simulink model "project 3 - RLS"  (R2018b)
settings: Solver=VariableStepAuto  StartTime=0.0  StopTime=1000  RelTol=1e-3
undefined symbols (not defined in the file): d, m, tmp
libraries: commchan3 x1
settings Model: Creator=DearUser  LastModifiedBy=DearUser

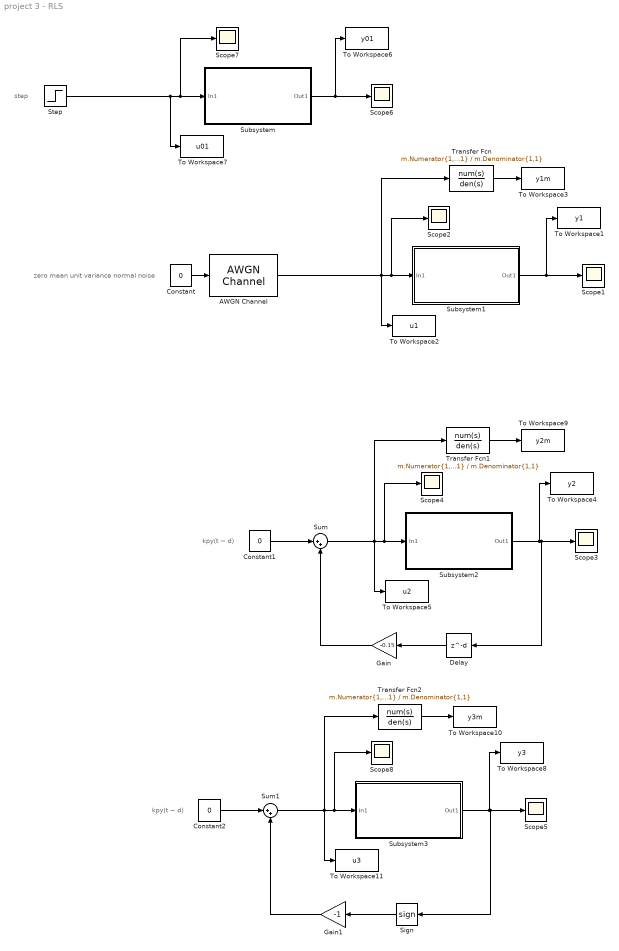
== system project 3 - RLS ==
  note: step
  note: zero mean unit variance normal noise
  note: kpy(t − d)
  note: kpy(t − d)
  AWGN Channel : commchan3/AWGN Channel  InputProcessing=Columns as channels (frame based)  seed=67  noiseMode=Variance from mask  EbNodB=10  EsNodB=10  SNRdB=10  bitsPerSym=1  Ps=1  Tsym=1  variance=1
      settings: SourceProductName=Communications Toolbox
  Constant : Constant  Value=0
  Constant1 : Constant  Value=0
  Constant2 : Constant  Value=0
  Delay : Delay  DelayLength=d
  Gain : Gain  Gain=-0.15
  Gain1 : Gain  Gain=-1
  Scope{1..8} (8 alike) : Scope
  Sign : Signum
  Step : Step  Time=100  SampleTime=0
  Subsystem : Subsystem  mask{sfcnParam1=tmp}
      mask prompts: sfcnParam1 "tmp:"
      mask help: Simulink:masks:GenSFuncDesc_MD
      mask Help: eval('feval(''rtwprivate'',''rtwhelpview'',''rtw_sfcn_block'')');
  Subsystem1 : Subsystem  mask{sfcnParam1=tmp}
      mask prompts: sfcnParam1 "tmp:"
      mask help: Simulink:masks:GenSFuncDesc_MD
      mask Help: eval('feval(''rtwprivate'',''rtwhelpview'',''rtw_sfcn_block'')');
  Subsystem2 : Subsystem  mask{sfcnParam1=tmp}
      mask prompts: sfcnParam1 "tmp:"
      mask help: Simulink:masks:GenSFuncDesc_MD
      mask Help: eval('feval(''rtwprivate'',''rtwhelpview'',''rtw_sfcn_block'')');
  Subsystem3 : Subsystem  mask{sfcnParam1=tmp}
      mask prompts: sfcnParam1 "tmp:"
      mask help: Simulink:masks:GenSFuncDesc_MD
      mask Help: eval('feval(''rtwprivate'',''rtwhelpview'',''rtw_sfcn_block'')');
  Sum : Sum  Inputs=|++
  Sum1 : Sum  Inputs=|++
  To Workspace1 : ToWorkspace  VariableName=y1  SaveFormat=Timeseries  SampleTime=-1
  To Workspace10 : ToWorkspace  VariableName=y3m  SaveFormat=Timeseries  SampleTime=-1
  To Workspace11 : ToWorkspace  VariableName=u3  SaveFormat=Timeseries  SampleTime=-1
  To Workspace2 : ToWorkspace  VariableName=u1  SaveFormat=Timeseries  SampleTime=-1
  To Workspace3 : ToWorkspace  VariableName=y1m  SaveFormat=Timeseries  SampleTime=-1
  To Workspace4 : ToWorkspace  VariableName=y2  SaveFormat=Timeseries  SampleTime=-1
  To Workspace5 : ToWorkspace  VariableName=u2  SaveFormat=Timeseries  SampleTime=-1
  To Workspace6 : ToWorkspace  VariableName=y01  SaveFormat=Timeseries  SampleTime=-1
  To Workspace7 : ToWorkspace  VariableName=u01  SaveFormat=Timeseries  SampleTime=-1
  To Workspace8 : ToWorkspace  VariableName=y3  SaveFormat=Timeseries  SampleTime=-1
  To Workspace9 : ToWorkspace  VariableName=y2m  SaveFormat=Timeseries  SampleTime=-1
  Transfer Fcn : TransferFcn  Numerator=m.Numerator{1,1}  Denominator=m.Denominator{1,1}
  Transfer Fcn1 : TransferFcn  Numerator=m.Numerator{1,1}  Denominator=m.Denominator{1,1}
  Transfer Fcn2 : TransferFcn  Numerator=m.Numerator{1,1}  Denominator=m.Denominator{1,1}
  wires:
  Subsystem/1(Out1) -> To Workspace6/1, Scope6/1
  Step/1 -> To Workspace7/1, Subsystem/1(In1), Scope7/1
  Constant/1 -> AWGN Channel/1
  AWGN Channel/1 -> To Workspace2/1, Subsystem1/1(In1), Scope2/1, Transfer Fcn/1
  Subsystem1/1(Out1) -> To Workspace1/1, Scope1/1
  Transfer Fcn/1 -> To Workspace3/1
  Constant1/1 -> Sum/1
  Delay/1 -> Gain/1
  Subsystem2/1(Out1) -> To Workspace4/1, Delay/1, Scope3/1
  Gain/1 -> Sum/2
  Transfer Fcn1/1 -> To Workspace9/1
  Sum/1 -> Transfer Fcn1/1, Subsystem2/1(In1), Scope4/1, To Workspace5/1
  Transfer Fcn2/1 -> To Workspace10/1
  Sign/1 -> Gain1/1
  Gain1/1 -> Sum1/2
  Subsystem3/1(Out1) -> To Workspace8/1, Sign/1, Scope5/1
  Constant2/1 -> Sum1/1
  Sum1/1 -> To Workspace11/1, Subsystem3/1(In1), Scope8/1, Transfer Fcn2/1

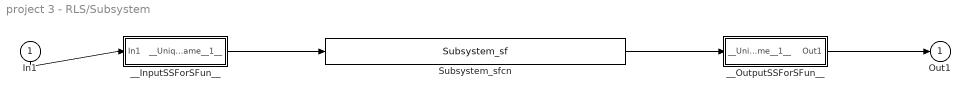
== system project 3 - RLS/Subsystem ==
  In1 : Inport
  Subsystem_sfcn : S-Function  FunctionName=Subsystem_sf  Parameters=sfcnParam1  SFunctionModules=""  SFunctionDeploymentMode=off  EnableBusSupport=off  mask{rtw_sf_name=Subsystem_sf, showVar=off, sfcnParam1=sfcnParam1}
      mask prompts: rtw_sf_name "Simulink:masks:GenSFuncName_MP"; showVar "Simulink:masks:GenSFuncShowModuleList_MP"; sfcnParam1 "tmp:"
      mask help: Simulink:masks:GenSFuncDesc_MD
      mask init:
      | displist = '';
      | if ~strcmp(get_param(gcb, 'FunctionName'), rtw_sf_name);
      |   set_param(gcb, 'FunctionName', rtw_sf_name);
      | end
      | % Check if we are generating code
      | rtw_mode = false;
      | if strcmpi(get_param(bdroot(gcb),'SimulationStatus'),'Initializing')
      | 	rtw_mode = strcmpi(get_param(bdroot(gcb),'BuildingRTWCode'),'on') && ...
      | 		~strcmpi(get_param(bdroot(gcb),'TargetStyle'),'SimulationTarget');
      | end
      | if showVar || rtw_mode
      | 	if exist('rtwsfunc') == 2 | exist('rtwsfunc') == 6
      | 		tmplist = rtwsfunc(rtw_sf_name,gcb);
      | 		tmplist = DAStudio.message('Simulink:masks:GenSFuncListOfModules_IC', tmplist);
      | 	elseif showVar
      | 		tmplist1 = DAStudio.message('Simulink:masks:GenSFuncListOfModules_IC', '');
      |         tmplist2 = DAStudio.message('Simulink:masks:GenSFuncNotLicensed_IC');
      |         tmplist = [tmplist1 tmplist2];
      |  	end
      | end
      | if showVar
      |   displist = tmplist;
      | end
      settings: CopyFcn=|
      | if ~strcmp(get_param(gcb,'Linkstatus'),'none') && ...
      | ~strcmp(get_param(gcb,'Linkstatus'),'implicit')
      |   set_param(gcb,'LinkStatus','none');
      | end
      mask Help: eval('feval(''rtwprivate'',''rtwhelpview'',''rtw_sfcn_block'')');
      mask Display:
      | port_label('input',1,'In1');
      | port_label('output',1,'Out1');
  __InputSSForSFun__ : Subsystem
  __OutputSSForSFun__ : Subsystem
  Out1 : Outport
  wires:
  In1/1 -> __InputSSForSFun__/1(In1)
  __InputSSForSFun__/1(__UniqueOutportName__1__) -> Subsystem_sfcn/1
  Subsystem_sfcn/1 -> __OutputSSForSFun__/1(__UniqueInportName__1__)
  __OutputSSForSFun__/1(Out1) -> Out1/1

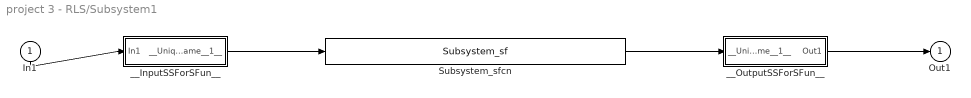
== system project 3 - RLS/Subsystem1 ==
  In1 : Inport
  Subsystem_sfcn : S-Function  FunctionName=Subsystem_sf  Parameters=sfcnParam1  SFunctionModules=""  SFunctionDeploymentMode=off  EnableBusSupport=off  mask{rtw_sf_name=Subsystem_sf, showVar=off, sfcnParam1=sfcnParam1}
      mask prompts: rtw_sf_name "Simulink:masks:GenSFuncName_MP"; showVar "Simulink:masks:GenSFuncShowModuleList_MP"; sfcnParam1 "tmp:"
      mask help: Simulink:masks:GenSFuncDesc_MD
      mask init: same as project 3 - RLS/Subsystem/Subsystem_sfcn
      settings: CopyFcn=|
      | if ~strcmp(get_param(gcb,'Linkstatus'),'none') && ...
      | ~strcmp(get_param(gcb,'Linkstatus'),'implicit')
      |   set_param(gcb,'LinkStatus','none');
      | end
      mask Help: eval('feval(''rtwprivate'',''rtwhelpview'',''rtw_sfcn_block'')');
      mask Display:
      | port_label('input',1,'In1');
      | port_label('output',1,'Out1');
  __InputSSForSFun__ : Subsystem
  __OutputSSForSFun__ : Subsystem
  Out1 : Outport
  wires:
  In1/1 -> __InputSSForSFun__/1(In1)
  __InputSSForSFun__/1(__UniqueOutportName__1__) -> Subsystem_sfcn/1
  Subsystem_sfcn/1 -> __OutputSSForSFun__/1(__UniqueInportName__1__)
  __OutputSSForSFun__/1(Out1) -> Out1/1

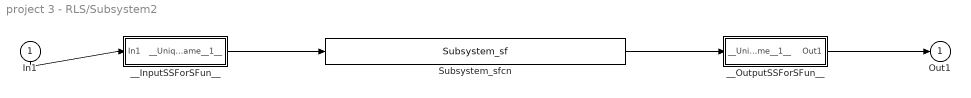
== system project 3 - RLS/Subsystem2 ==
  In1 : Inport
  Subsystem_sfcn : S-Function  FunctionName=Subsystem_sf  Parameters=sfcnParam1  SFunctionModules=""  SFunctionDeploymentMode=off  EnableBusSupport=off  mask{rtw_sf_name=Subsystem_sf, showVar=off, sfcnParam1=sfcnParam1}
      mask prompts: rtw_sf_name "Simulink:masks:GenSFuncName_MP"; showVar "Simulink:masks:GenSFuncShowModuleList_MP"; sfcnParam1 "tmp:"
      mask help: Simulink:masks:GenSFuncDesc_MD
      mask init: same as project 3 - RLS/Subsystem/Subsystem_sfcn
      settings: CopyFcn=|
      | if ~strcmp(get_param(gcb,'Linkstatus'),'none') && ...
      | ~strcmp(get_param(gcb,'Linkstatus'),'implicit')
      |   set_param(gcb,'LinkStatus','none');
      | end
      mask Help: eval('feval(''rtwprivate'',''rtwhelpview'',''rtw_sfcn_block'')');
      mask Display:
      | port_label('input',1,'In1');
      | port_label('output',1,'Out1');
  __InputSSForSFun__ : Subsystem
  __OutputSSForSFun__ : Subsystem
  Out1 : Outport
  wires:
  In1/1 -> __InputSSForSFun__/1(In1)
  __InputSSForSFun__/1(__UniqueOutportName__1__) -> Subsystem_sfcn/1
  Subsystem_sfcn/1 -> __OutputSSForSFun__/1(__UniqueInportName__1__)
  __OutputSSForSFun__/1(Out1) -> Out1/1

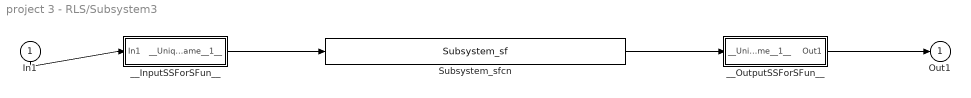
== system project 3 - RLS/Subsystem3 ==
  In1 : Inport
  Subsystem_sfcn : S-Function  FunctionName=Subsystem_sf  Parameters=sfcnParam1  SFunctionModules=""  SFunctionDeploymentMode=off  EnableBusSupport=off  mask{rtw_sf_name=Subsystem_sf, showVar=off, sfcnParam1=sfcnParam1}
      mask prompts: rtw_sf_name "Simulink:masks:GenSFuncName_MP"; showVar "Simulink:masks:GenSFuncShowModuleList_MP"; sfcnParam1 "tmp:"
      mask help: Simulink:masks:GenSFuncDesc_MD
      mask init: same as project 3 - RLS/Subsystem/Subsystem_sfcn
      settings: CopyFcn=|
      | if ~strcmp(get_param(gcb,'Linkstatus'),'none') && ...
      | ~strcmp(get_param(gcb,'Linkstatus'),'implicit')
      |   set_param(gcb,'LinkStatus','none');
      | end
      mask Help: eval('feval(''rtwprivate'',''rtwhelpview'',''rtw_sfcn_block'')');
      mask Display:
      | port_label('input',1,'In1');
      | port_label('output',1,'Out1');
  __InputSSForSFun__ : Subsystem
  __OutputSSForSFun__ : Subsystem
  Out1 : Outport
  wires:
  In1/1 -> __InputSSForSFun__/1(In1)
  __InputSSForSFun__/1(__UniqueOutportName__1__) -> Subsystem_sfcn/1
  Subsystem_sfcn/1 -> __OutputSSForSFun__/1(__UniqueInportName__1__)
  __OutputSSForSFun__/1(Out1) -> Out1/1

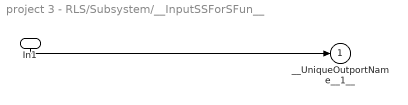
== system project 3 - RLS/Subsystem/__InputSSForSFun__ ==
  In1 : Inport
  __UniqueOutportName__1__ : Outport
  wires:
  In1/1 -> __UniqueOutportName__1__/1

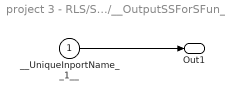
== system project 3 - RLS/Subsystem/__OutputSSForSFun__ ==
  __UniqueInportName__1__ : Inport
  Out1 : Outport
  wires:
  __UniqueInportName__1__/1 -> Out1/1

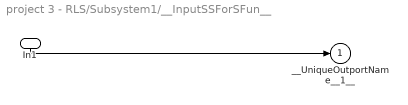
== system project 3 - RLS/Subsystem1/__InputSSForSFun__ ==
  In1 : Inport
  __UniqueOutportName__1__ : Outport
  wires:
  In1/1 -> __UniqueOutportName__1__/1

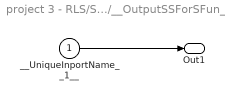
== system project 3 - RLS/Subsystem1/__OutputSSForSFun__ ==
  __UniqueInportName__1__ : Inport
  Out1 : Outport
  wires:
  __UniqueInportName__1__/1 -> Out1/1

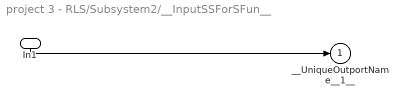
== system project 3 - RLS/Subsystem2/__InputSSForSFun__ ==
  In1 : Inport
  __UniqueOutportName__1__ : Outport
  wires:
  In1/1 -> __UniqueOutportName__1__/1

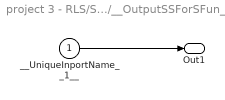
== system project 3 - RLS/Subsystem2/__OutputSSForSFun__ ==
  __UniqueInportName__1__ : Inport
  Out1 : Outport
  wires:
  __UniqueInportName__1__/1 -> Out1/1

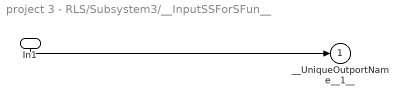
== system project 3 - RLS/Subsystem3/__InputSSForSFun__ ==
  In1 : Inport
  __UniqueOutportName__1__ : Outport
  wires:
  In1/1 -> __UniqueOutportName__1__/1

== system project 3 - RLS/Subsystem3/__OutputSSForSFun__ ==
  __UniqueInportName__1__ : Inport
  Out1 : Outport
  wires:
  __UniqueInportName__1__/1 -> Out1/1
